simulink model "FCC"  (R2021b)
settings: Solver=VariableStepAuto  StartTime=0.0  StopTime=10.0  RelTol=1e-3
settings Model: Creator=ACH  LastModifiedBy=ACH

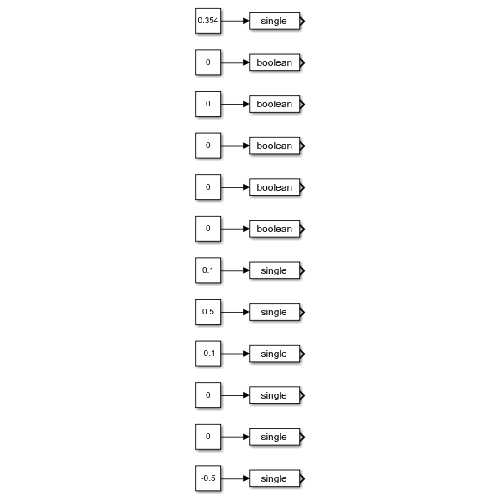
[thumbnail: Simulink's stored preview of the top-level diagram]
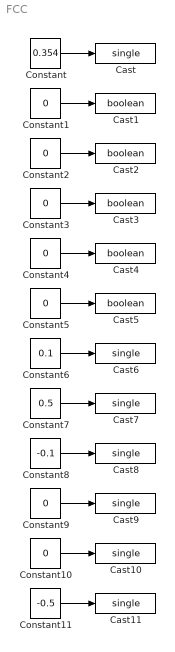
== system FCC ==
  Cast{,6..11} (7 alike) : DataTypeConversion  OutDataTypeStr=single
  Cast{1..5} (5 alike) : DataTypeConversion  OutDataTypeStr=boolean
  Constant : Constant  Value=0.354
  Constant{1..5,9..10} (7 alike) : Constant  Value=0
  Constant11 : Constant  Value=-0.5
  Constant6 : Constant  Value=0.1
  Constant7 : Constant  Value=0.5
  Constant8 : Constant  Value=-0.1
  wires:
  Constant/1 -> Cast/1
  Constant1/1 -> Cast1/1
  Constant2/1 -> Cast2/1
  Constant3/1 -> Cast3/1
  Constant4/1 -> Cast4/1
  Constant5/1 -> Cast5/1
  Constant6/1 -> Cast6/1
  Constant7/1 -> Cast7/1
  Constant8/1 -> Cast8/1
  Constant9/1 -> Cast9/1
  Constant10/1 -> Cast10/1
  Constant11/1 -> Cast11/1
